simulink model "fft_synthesis"  (R2020b)
settings: Solver=FixedStepDiscrete  StartTime=0.0  StopTime=0.01  RelTol=1e-3
undefined symbols (not defined in the file or in its folder): mp
libraries: hdlsllib x7, simulink x1, dsphdlxfrm x1
settings Model: DataTypeOverride=Off  Creator=Ross  LastModifiedBy=wickh
settings DataIOCC: SaveOutput=off  SaveTime=off  ReturnWorkspaceOutputs=off
settings OptimizationCC: BlockReduction=off  ConditionallyExecuteInputs=off  DefaultParameterBehavior=Inlined
settings DebuggingCC: ReadBeforeWriteMsg=DisableAll  WriteAfterWriteMsg=DisableAll  WriteAfterReadMsg=DisableAll  AlgebraicLoopMsg=error  MultiTaskDSMMsg=none  SingleTaskRateTransMsg=error  PregeneratedLibrarySubsystemCodeDiagnostic=none  ArithmeticOperatorsInVariantConditions=warning
settings HardwareCC: ProdBitPerPointer=32  ProdBitPerSizeT=32  ProdBitPerPtrDiffT=32  ProdLargestAtomicFloat=None  ProdIntDivRoundTo=Undefined  ProdEndianess=Unspecified  ProdWordSize=32  ProdHWDeviceType=ASIC/FPGA->ASIC/FPGA  TargetBitPerPointer=64  TargetBitPerSizeT=64  TargetBitPerPtrDiffT=64  TargetLongLongMode=on  TargetIntDivRoundTo=Zero  TargetEndianess=LittleEndian  TargetWordSize=64  TargetHWDeviceType=Custom Processor->MATLAB Host Computer  ProdEqTarget=off
settings ModelReferenceCC: UpdateModelReferenceTargets=IfOutOfDate
settings SFSimCC: SFSimEcho=off  SimUseLocalCustomCode=off  CustomCodeUndefinedFunction=UseInterfaceOnly
settings RTWCC: RTWUseLocalCustomCode=off

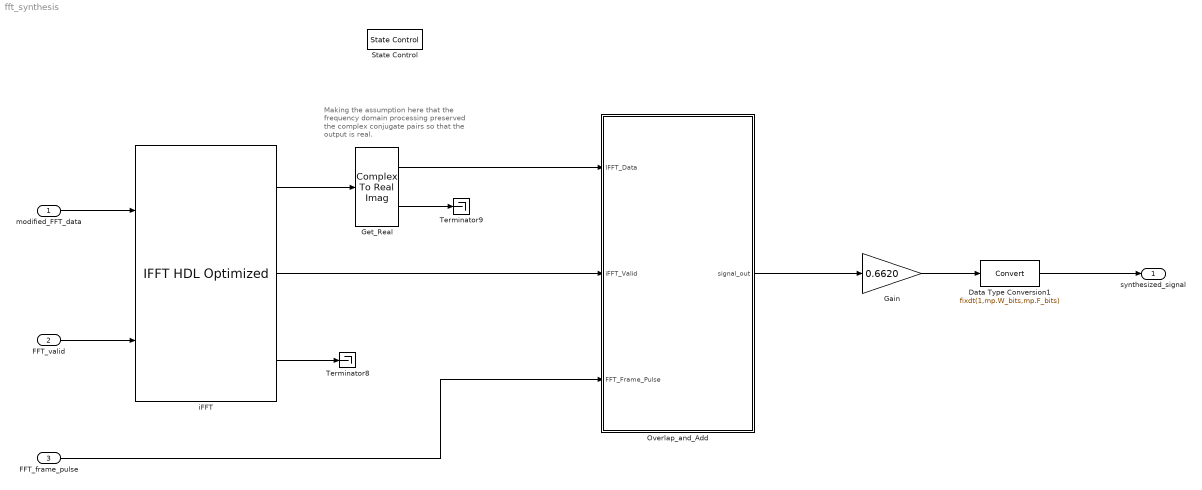
== system fft_synthesis ==
  note: Making the assumption here
      | that the frequency domain processing
      | preserved the complex conjugate pairs
      | so that the output is real.
  modified_FFT_data : Inport  OutDataTypeStr=fixdt(1,31,23)  PortDimensions=1  SampleTime=[1.6276041666666666e-07,0]
      settings: SignalType=complex
  FFT_valid : Inport  Port=2  OutDataTypeStr=boolean  PortDimensions=1  SampleTime=[1.6276041666666666e-07,0]
  FFT_frame_pulse : Inport  Port=3  OutDataTypeStr=boolean  PortDimensions=1  SampleTime=[1.6276041666666666e-07,0]
  Data Type Conversion1 : DataTypeConversion  OutDataTypeStr=fixdt(1,mp.W_bits,mp.F_bits)
  Gain : Gain  Gain=0.6620
  Get_Real : ComplexToRealImag
  Overlap_and_Add : Subsystem
  State Control : StateControl  StateControl=Synchronous
  Terminator8 : Terminator
  Terminator9 : Terminator
  iFFT : dsphdlxfrm/IFFT HDL Optimized  FFTLength=mp.FFT_size  Architecture=Burst Radix 2  ComplexMultiplication=Use 4 multipliers and 2 adders  BitReversedOutput=off  BitReversedInput=off  Normalize=on  SimulateUsing=Code generation  RoundingMethod=Floor  ResetInputPort=off  StartOutputPort=off  EndOutputPort=off
      settings: SourceProductBaseCode=DS
  synthesized_signal : Outport  OutDataTypeStr=fixdt(1,24,23)  PortDimensions=1  VectorParamsAs1DForOutWhenUnconnected=off
  wires:
  iFFT/3 -> Terminator8/1
  iFFT/2 -> Overlap_and_Add/2(iFFT_Valid)
  Get_Real/1 -> Overlap_and_Add/1(IFFT_Data)
  modified_FFT_data/1 -> iFFT/1
  Data Type Conversion1/1 -> synthesized_signal/1
  iFFT/1 -> Get_Real/1
  Get_Real/2 -> Terminator9/1
  FFT_valid/1 -> iFFT/2
  FFT_frame_pulse/1 -> Overlap_and_Add/3(FFT_Frame_Pulse)
  Overlap_and_Add/1(signal_out) -> Gain/1
  Gain/1 -> Data Type Conversion1/1

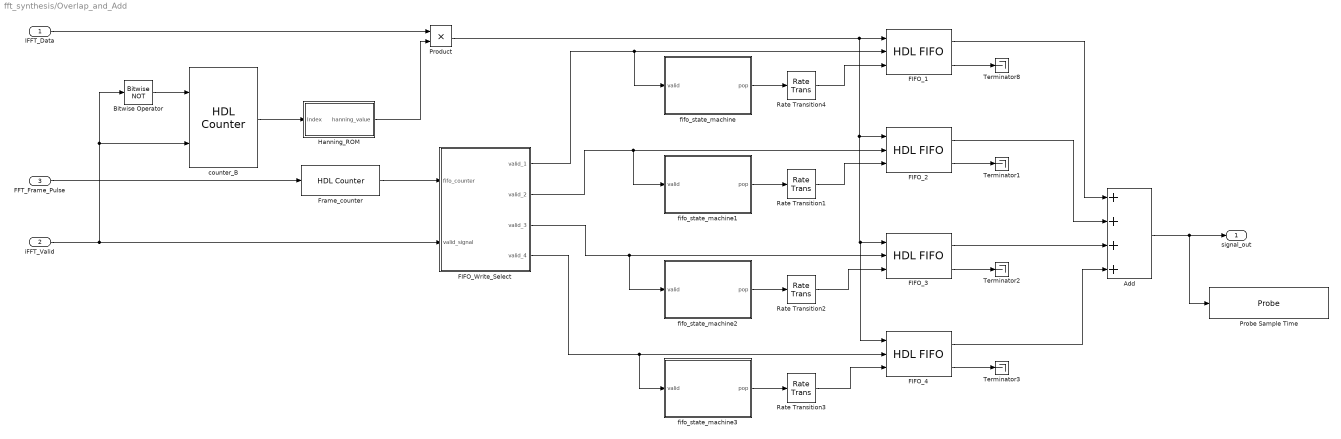
== system fft_synthesis/Overlap_and_Add ==
  IFFT_Data : Inport
  iFFT_Valid : Inport  Port=2
  FFT_Frame_Pulse : Inport  Port=3
  Add : Sum  Inputs=4
  Bitwise Operator : simulink/Logic and Bit Operations/Bitwise Operator  logicop=NOT  UseBitMask=off  BitMask=bin2dec('11011001')  BitMaskRealWorld=Stored Integer
  FIFO_{1..4} (4 alike) : hdlsllib/HDL RAMs/HDL FIFO  fifo_size=mp.FFT_size  mode=Classic  ratio=mp.SysRate_Upsample_Factor  push_msg=Warning  pop_msg=Warning  show_empty=off  show_full=on  show_num=off  LabelModeActiveChoice_Mode=Classic
      settings: SourceProductBaseCode=SL
  FIFO_Write_Select : MATLAB Function  TreatAsAtomicUnit=on
  Frame_counter : hdlsllib/Sources/HDL Counter  CountType=Free running  CountInit=2  CountStep=1  CountMax=1024  CountFromType=Initial value  CountFrom=2  CountResetPort=off  CountLoadPort=off  CountEnbPort=on  CountDirPort=off  CountDataType=Unsigned  CountWordLen=2  CountFracLen=0  CountSampTime=1
  Hanning_ROM : Subsystem
  Probe Sample Time : Probe  ProbeWidth=off  ProbeComplexSignal=off
  Product : Product  OutDataTypeStr=Inherit: Same as first input
  Rate Transition{1..4} (4 alike) : RateTransition  OutPortSampleTimeOpt=Multiple of input port sample time  OutPortSampleTimeMultiple=mp.SysRate_Upsample_Factor
  Terminator{1..3,8} (4 alike) : Terminator
  counter_B : hdlsllib/Sources/HDL Counter  CountType=Count limited  CountInit=0  CountStep=1  CountMax=mp.FFT_size  CountFromType=Initial value  CountFrom=0  CountResetPort=on  CountLoadPort=off  CountEnbPort=on  CountDirPort=off  CountDataType=Unsigned  CountWordLen=mp.DPRAM1_address_size  CountFracLen=0  CountSampTime=1
  fifo_state_machine : MATLAB Function  TreatAsAtomicUnit=on
  fifo_state_machine1 : MATLAB Function  TreatAsAtomicUnit=on
  fifo_state_machine2 : MATLAB Function  TreatAsAtomicUnit=on
  fifo_state_machine3 : MATLAB Function  TreatAsAtomicUnit=on
  signal_out : Outport  VectorParamsAs1DForOutWhenUnconnected=off
  wires:
  Product/1 -> FIFO_1/1, FIFO_2/1, FIFO_3/1, FIFO_4/1
  Rate Transition3/1 -> FIFO_4/3
  fifo_state_machine3/1(pop) -> Rate Transition3/1
  Rate Transition2/1 -> FIFO_3/3
  fifo_state_machine2/1(pop) -> Rate Transition2/1
  Rate Transition1/1 -> FIFO_2/3
  fifo_state_machine1/1(pop) -> Rate Transition1/1
  FIFO_1/2 -> Terminator8/1
  Rate Transition4/1 -> FIFO_1/3
  fifo_state_machine/1(pop) -> Rate Transition4/1
  counter_B/1 -> Hanning_ROM/1(Index)
  Hanning_ROM/1(hanning_value) -> Product/2
  IFFT_Data/1 -> Product/1
  iFFT_Valid/1 -> FIFO_Write_Select/2(valid_signal), Bitwise Operator/1, counter_B/2
  Bitwise Operator/1 -> counter_B/1
  FIFO_3/2 -> Terminator2/1
  FIFO_2/2 -> Terminator1/1
  FIFO_4/2 -> Terminator3/1
  Frame_counter/1 -> FIFO_Write_Select/1(fifo_counter)
  FIFO_Write_Select/2(valid_2) -> FIFO_2/2, fifo_state_machine1/1(valid)
  FIFO_Write_Select/1(valid_1) -> FIFO_1/2, fifo_state_machine/1(valid)
  FIFO_4/1 -> Add/4
  FIFO_Write_Select/4(valid_4) -> FIFO_4/2, fifo_state_machine3/1(valid)
  FIFO_Write_Select/3(valid_3) -> FIFO_3/2, fifo_state_machine2/1(valid)
  FIFO_2/1 -> Add/2
  FFT_Frame_Pulse/1 -> Frame_counter/1
  FIFO_3/1 -> Add/3
  FIFO_1/1 -> Add/1
  Add/1 -> Probe Sample Time/1, signal_out/1

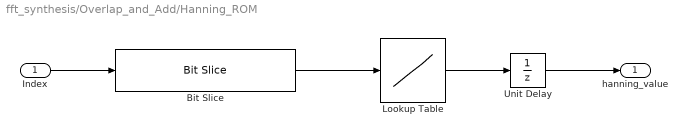
== system fft_synthesis/Overlap_and_Add/Hanning_ROM ==
  Index : Inport
  Bit Slice : hdlsllib/Logic and Bit Operations/Bit Slice  lidx=log2(mp.FFT_size) - 1  ridx=0
      settings: SourceProductBaseCode=SL
  Lookup Table : Lookup_n-D  NumberOfTableDimensions=1  BreakpointsForDimension1=[0:mp.FFT_size-1]  IndexSearchMethod=Evenly spaced points  Table=hanning(mp.FFT_size)  InterpMethod=Flat  ExtrapMethod=Clip  DiagnosticForOutOfRangeInput=Error  UseLastTableValue=on  OutDataTypeStr=fixdt(1,24,22)  RndMeth=Simplest  InputSameDT=on
  Unit Delay : UnitDelay  SampleTime=-1  HasFrameUpgradeWarning=on
  hanning_value : Outport  VectorParamsAs1DForOutWhenUnconnected=off
  wires:
  Bit Slice/1 -> Lookup Table/1
  Lookup Table/1 -> Unit Delay/1
  Index/1 -> Bit Slice/1
  Unit Delay/1 -> hanning_value/1

== matlab function fft_synthesis/Overlap_and_Add/fifo_state_machine1 ==
  data: valid input; pop output
function pop = fifo_state_machine(valid)
%#codegen

state_valid_low = fi(0, 0, 2, 0);
state_valid_high = fi(1, 0, 2, 0);
state_assert_pop = fi(2, 0, 2, 0);

persistent current_state;
if isempty(current_state)
    current_state = state_valid_low;
end

switch(current_state)
    case state_valid_low

        pop = false;
        
        if valid
            current_state = state_valid_high;
        else
            current_state = state_valid_low;
        end
        
    case state_valid_high
        
        pop = false;
        
        if valid
            current_state = state_valid_high;
        else
            current_state = state_assert_pop;
        end
        
    case state_assert_pop
        
        pop = true;
        
        current_state = state_assert_pop;
        
    otherwise
        
        pop = false;
        
end

== matlab function fft_synthesis/Overlap_and_Add/fifo_state_machine2 ==
  data: valid input; pop output
function pop = fifo_state_machine(valid)
%#codegen

state_valid_low = fi(0, 0, 2, 0);
state_valid_high = fi(1, 0, 2, 0);
state_assert_pop = fi(2, 0, 2, 0);

persistent current_state;
if isempty(current_state)
    current_state = state_valid_low;
end

switch(current_state)
    case state_valid_low

        pop = false;
        
        if valid
            current_state = state_valid_high;
        else
            current_state = state_valid_low;
        end
        
    case state_valid_high
        
        pop = false;
        
        if valid
            current_state = state_valid_high;
        else
            current_state = state_assert_pop;
        end
        
    case state_assert_pop
        
        pop = true;
        
        current_state = state_assert_pop;
        
    otherwise
        
        pop = false;
        
end

== matlab function fft_synthesis/Overlap_and_Add/fifo_state_machine3 ==
  data: valid input; pop output
function pop = fifo_state_machine(valid)
%#codegen

state_valid_low = fi(0, 0, 2, 0);
state_valid_high = fi(1, 0, 2, 0);
state_assert_pop = fi(2, 0, 2, 0);

persistent current_state;
if isempty(current_state)
    current_state = state_valid_low;
end

switch(current_state)
    case state_valid_low

        pop = false;
        
        if valid
            current_state = state_valid_high;
        else
            current_state = state_valid_low;
        end
        
    case state_valid_high
        
        pop = false;
        
        if valid
            current_state = state_valid_high;
        else
            current_state = state_assert_pop;
        end
        
    case state_assert_pop
        
        pop = true;
        
        current_state = state_assert_pop;
        
    otherwise
        
        pop = false;
        
end

== matlab function fft_synthesis/Overlap_and_Add/FIFO_Write_Select ==
  data: fifo_counter input; valid_1 output; valid_signal input; valid_2 output; valid_3 output; valid_4 output
function [valid_1, valid_2, valid_3, valid_4] = fcn(fifo_counter, valid_signal)
%#codegen



switch fifo_counter
    case 0
        valid_1 = valid_signal;
        valid_2 = false;
        valid_3 = false;
        valid_4 = false;
    case 1
        valid_1 = false;
        valid_2 = valid_signal;
        valid_3 = false;
        valid_4 = false;
    case 2
        valid_1 = false;
        valid_2 = false;
        valid_3 = valid_signal;
        valid_4 = false;
    case 3
        valid_1 = false;
        valid_2 = false;
        valid_3 = false;
        valid_4 = valid_signal;
    otherwise
        valid_1 = false;
        valid_2 = false;
        valid_3 = false;
        valid_4 = false;
       
end

== matlab function fft_synthesis/Overlap_and_Add/fifo_state_machine ==
  data: valid input; pop output
function pop = fifo_state_machine(valid)
%#codegen

state_valid_low = fi(0, 0, 2, 0);
state_valid_high = fi(1, 0, 2, 0);
state_assert_pop = fi(2, 0, 2, 0);

persistent current_state;
if isempty(current_state)
    current_state = state_valid_low;
end

switch(current_state)
    case state_valid_low

        pop = false;
        
        if valid
            current_state = state_valid_high;
        else
            current_state = state_valid_low;
        end
        
    case state_valid_high
        
        pop = false;
        
        if valid
            current_state = state_valid_high;
        else
            current_state = state_assert_pop;
        end
        
    case state_assert_pop
        
        pop = true;
        
        current_state = state_assert_pop;
        
    otherwise
        
        pop = false;
        
end
